simulink model "sampleModel1602"  (R2023a)
settings: Solver=VariableStepAuto  StartTime=0.0  StopTime=10.0  RelTol=1e-3
libraries: hdlsllib x5, simulink x1
settings Model: Creator=user1  LastModifiedBy=user1

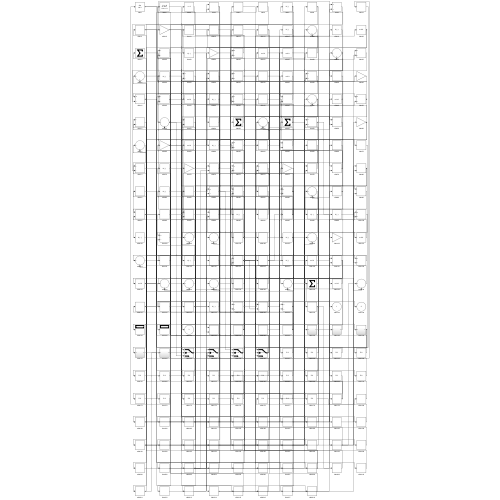
[thumbnail: Simulink's stored preview of the top-level diagram]
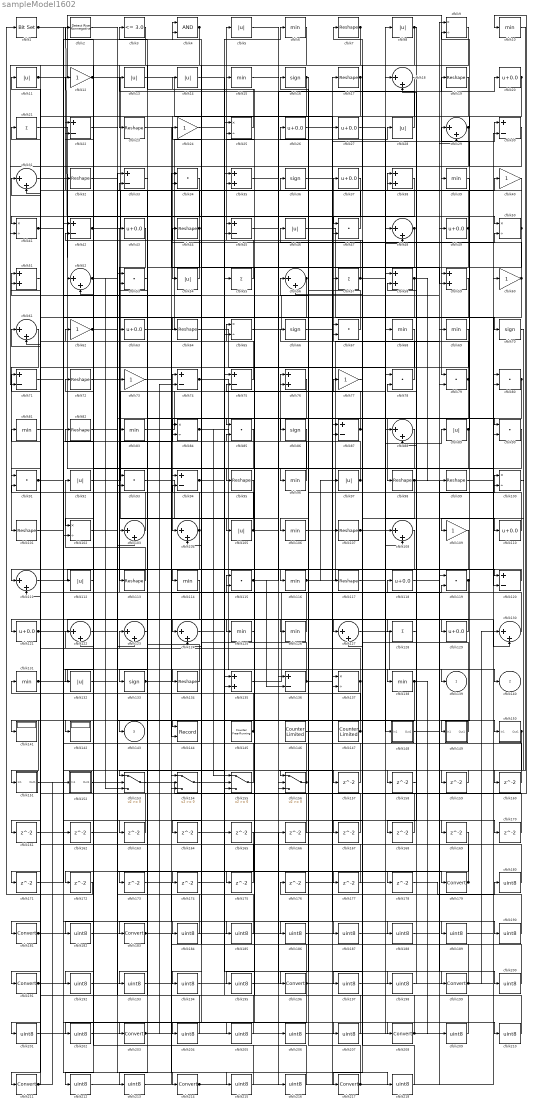
== system sampleModel1602 ==
  cfblk1 : simulink/Logic and Bit Operations/Bit Set  iBit=0
      settings: LibrarySourceBlock=|
      | hdlsllib/Logic and Bit
      | Operations/Bit Set
  cfblk{6,10,15,39,68..69,81,83,96,106,114,116,125..126,131,138} (16 alike) : MinMax
  cfblk{9,25,41,50,65,84,100,102,137} (9 alike) : Product  Inputs=*/  RndMeth=Zero  SaturateOnIntegerOverflow=on
  cfblk{7,17,19,23,32,44,64,72,82,95,98..99,101,107,113,117,134} (17 alike) : Reshape
  cfblk{18,29,31,48,52,56,61,88,103..104,108,111,122..124,127,130} (17 alike) : Sum  Inputs=|++
  cfblk{5,8,11,13..14,28,46,54,89,92,97,105,112,132} (14 alike) : Abs  SaturateOnIntegerOverflow=off
  cfblk{12,24,40,60,62,73,77,109} (8 alike) : Gain
  cfblk{20,26..27,37,43,49,63,110,118,121,129} (11 alike) : Bias  Bias=0.0  SaturateOnIntegerOverflow=off
  cfblk{34,47,53,67,78..80,85,90..91,93,115,119} (13 alike) : DotProduct  OutDataTypeStr=Inherit: Inherit via internal rule
  cfblk{22,30,33,42,45,71,74..75,87,94,120,136} (12 alike) : Sum  Inputs=+-
  cfblk{21,55,57,128} (4 alike) : Sum  Inputs=+
  cfblk{16,36,66,70,86,133} (6 alike) : Signum
  cfblk{35,38,51,58..59,76,135} (7 alike) : Sum
  cfblk141 : Display
  cfblk142 : Display
  cfblk144 : Record  FileSettingsInternal="{\"entries\":[{\"content\":{\"excelSettings\":{\"content\":{},\"type\":\"Streamout.ExcelSettings\"}},\"type\":\"Streamout.FileSettingStorage\",\"uuid\":\"\"}],\"packageUris\":[\"http:\\/\\/schema.mathworks.com\\/mf0\\/streamout_blocks\\/R2020a\"],\"version\":\"1.0\"}"  Layout=[1 1]  SignalsInternal="{\"entries\":[{\"content\":{\"signals\":[{\"content\":{\"blockPath\":[],\"dimensions\":[1],\"domain\":\"\",\"lineColor\":\"#a2142f\",\"plots\":[1],\"port\":1,\"signalID\":2228,\"signalName\":\"XY Graph:1\"},\"type\":\"RecordBlkView.Signal\",\"uuid\":\"\"},{\"content\":{\"blockPath\":[],\"dimensions\":[1],\"domain\":\"\",\"lineColor\":\"#139fff\",\"plots\":[1],\"port\":2,\"signalID\":2231,\"signalName\":\"XY Graph:2\"},\"type\":\"RecordBlkView.Signal\",\"uuid\":\"\"}]},\"type\":\"RecordBlkView.InputSignals\",\"uuid\":\"\"}],\"packageUris\":[\"http:\\/\\/schema.mathworks.com\\/mf0\\/streamout_blocks\\/R2020a\"],\"version\":\"1.0\"}"  VisualizationBindings="{\"xyplotplugin\":{\"info\":[{\"series\":[{\"bindingParametersList\":[{\"parameter\":\"X-Axis\",\"signalID\":2228,\"signalName\":\"XY Graph:1\"},{\"parameter\":\"Y-Axis\",\"signalID\":2231,\"signalName\":\"XY Graph:2\"}],\"seriesID\":22557}],\"subplotID\":1}]}}"  CompatibilityTag=XY  st=-1
  cfblk145 : hdlsllib/Sources/Counter Free-Running  NumBits=16  tsamp=-1
  cfblk146 : hdlsllib/Sources/Counter Limited  uplimit=7  tsamp=-1
  cfblk147 : hdlsllib/Sources/Counter Limited  uplimit=7  tsamp=-1
  cfblk148 : Subsystem
      settings: LibrarySourceBlock=|
      | hdlsllib/Ports &
      | Subsystems/Subsystem
  cfblk149 : Subsystem
      settings: LibrarySourceBlock=|
      | hdlsllib/Ports &
      | Subsystems/Subsystem
  cfblk150 : Subsystem
      settings: LibrarySourceBlock=|
      | hdlsllib/Ports &
      | Subsystems/Subsystem
  cfblk151 : Subsystem
      settings: LibrarySourceBlock=|
      | hdlsllib/Ports &
      | Subsystems/Subsystem
  cfblk152 : Subsystem
      settings: LibrarySourceBlock=|
      | hdlsllib/Ports &
      | Subsystems/Subsystem
  cfblk{153..156} (4 alike) : Switch  SaturateOnIntegerOverflow=off  InputSameDT=off
  cfblk{157..178} (22 alike) : Delay  SampleTime=1
  cfblk{179,181,183,191,196,199,203,208,211,214,217} (11 alike) : DataTypeConversion  SaturateOnIntegerOverflow=off  RndMeth=Floor
  cfblk{180,182,184..190,192..195,197..198,200..202,204..207,209..210,212..213,215..216,218} (29 alike) : DataTypeConversion  OutDataTypeStr=uint8  SaturateOnIntegerOverflow=off  RndMeth=Floor
  cfblk2 : hdlsllib/Logic and Bit Operations/Detect Rise Nonnegative  vinit=0  OutDataTypeStr=boolean
  cfblk3 : hdlsllib/Logic and Bit Operations/Compare To Constant  relop=<=  const=3.0  OutDataTypeStr=boolean
  cfblk4 : Logic  AllPortsSameDT=off  OutDataTypeStr=boolean
  cfblk139 : Outport  VectorParamsAs1DForOutWhenUnconnected=off
  cfblk140 : Outport  Port=2  VectorParamsAs1DForOutWhenUnconnected=off
  cfblk143 : Outport  Port=3  VectorParamsAs1DForOutWhenUnconnected=off
  wires:
  cfblk33/1 -> cfblk203/1
  cfblk127/1 -> cfblk139/1
  cfblk8/1 -> cfblk167/1, cfblk168/1
  cfblk135/1 -> cfblk118/1
  cfblk84/1 -> cfblk120/1, cfblk155/1
  cfblk119/1 -> cfblk131/1, cfblk174/1, cfblk201/1
  cfblk117/1 -> cfblk89/1
  cfblk57/1 -> cfblk5/1, cfblk110/1
  cfblk74/1 -> cfblk140/1, cfblk4/1
  cfblk12/1 -> cfblk105/1, cfblk100/2
  cfblk42/1 -> cfblk38/1, cfblk102/1
  cfblk53/1 -> cfblk183/1
  cfblk52/1 -> cfblk123/2, cfblk153/3
  cfblk63/1 -> cfblk28/1
  cfblk21/1 -> cfblk96/1
  cfblk126/1 -> cfblk43/1
  cfblk11/1 -> cfblk79/1, cfblk155/3
  cfblk43/1 -> cfblk113/1
  cfblk64/1 -> cfblk148/1(In1)
  cfblk19/1 -> cfblk54/1
  cfblk38/1 -> cfblk126/1
  cfblk61/1 -> cfblk101/1
  cfblk20/1 -> cfblk41/1, cfblk39/1
  cfblk70/1 -> cfblk109/1
  cfblk97/1 -> cfblk74/1, cfblk83/1
  cfblk78/1 -> cfblk37/1
  cfblk125/1 -> cfblk45/1
  cfblk24/1 -> cfblk55/1
  cfblk96/1 -> cfblk76/1
  cfblk154/1 -> cfblk199/1
  cfblk89/1 -> cfblk29/1, cfblk94/1
  cfblk7/1 -> cfblk114/1, cfblk173/1
  cfblk69/1 -> cfblk181/1
  cfblk128/1 -> cfblk58/2
  cfblk39/1 -> cfblk149/1(In1)
  cfblk1/1 -> cfblk52/1, cfblk65/2
  cfblk79/1 -> cfblk98/1, cfblk26/1, cfblk66/1
  cfblk129/1 -> cfblk125/1
  cfblk9/1 -> cfblk23/1
  cfblk76/1 -> cfblk104/1
  cfblk48/1 -> cfblk95/1, cfblk204/1
  cfblk35/1 -> cfblk208/1
  cfblk121/1 -> cfblk124/1, cfblk84/2, cfblk4/2
  cfblk146/1 -> cfblk27/1
  cfblk95/1 -> cfblk103/1
  cfblk40/1 -> cfblk38/2
  cfblk67/1 -> cfblk16/1
  cfblk14/1 -> cfblk179/1
  cfblk31/1 -> cfblk47/1
  cfblk80/1 -> cfblk153/1, cfblk158/1
  cfblk150/1(Out1) -> cfblk195/1, cfblk213/1
  cfblk108/1 -> cfblk191/1
  cfblk2/1 -> cfblk103/2
  cfblk4/1 -> cfblk141/1, cfblk192/1
  cfblk138/1 -> cfblk155/2, cfblk209/1
  cfblk111/1 -> cfblk116/1
  cfblk107/1 -> cfblk129/1, cfblk197/1
  cfblk149/1(Out1) -> cfblk56/2
  cfblk94/1 -> cfblk24/1, cfblk6/1
  cfblk60/1 -> cfblk46/1, cfblk87/2, cfblk171/1
  cfblk37/1 -> cfblk91/1
  cfblk47/1 -> cfblk12/1
  cfblk72/1 -> cfblk90/1
  cfblk105/1 -> cfblk136/1, cfblk72/1
  cfblk102/1 -> cfblk128/1
  cfblk147/1 -> cfblk44/1, cfblk84/1
  cfblk17/1 -> cfblk45/2, cfblk143/1
  cfblk93/1 -> cfblk156/2
  cfblk115/1 -> cfblk20/1, cfblk136/2, cfblk130/2, cfblk178/1, cfblk198/1
  cfblk75/1 -> cfblk31/2
  cfblk28/1 -> cfblk13/1
  cfblk136/1 -> cfblk19/1, cfblk51/2
  cfblk22/1 -> cfblk67/2
  cfblk30/1 -> cfblk59/1
  cfblk27/1 -> cfblk70/1
  cfblk50/1 -> cfblk7/1, cfblk135/2
  cfblk153/1 -> cfblk10/1
  cfblk131/1 -> cfblk134/1, cfblk57/1
  cfblk92/1 -> cfblk17/1
  cfblk123/1 -> cfblk93/1
  cfblk56/1 -> cfblk104/2, cfblk64/1, cfblk144/2
  cfblk26/1 -> cfblk50/1
  cfblk44/1 -> cfblk21/1, cfblk193/1
  cfblk25/1 -> cfblk3/1
  cfblk66/1 -> cfblk30/1
  cfblk113/1 -> cfblk92/1
  cfblk116/1 -> cfblk9/1, cfblk97/1
  cfblk77/1 -> cfblk217/1
  cfblk134/1 -> cfblk63/1
  cfblk88/1 -> cfblk196/1
  cfblk86/1 -> cfblk133/1
  cfblk118/1 -> cfblk100/1
  cfblk73/1 -> cfblk50/2
  cfblk54/1 -> cfblk42/2
  cfblk106/1 -> cfblk48/1
  cfblk130/1 -> cfblk71/1
  cfblk46/1 -> cfblk120/2
  cfblk109/1 -> cfblk156/3
  cfblk91/1 -> cfblk138/1, cfblk153/2
  cfblk99/1 -> cfblk90/2
  cfblk13/1 -> cfblk107/1
  cfblk3/1 -> cfblk41/2
  cfblk58/1 -> cfblk86/1, cfblk99/1
  cfblk29/1 -> cfblk71/2, cfblk9/2, cfblk142/1
  cfblk103/1 -> cfblk81/1
  cfblk155/1 -> cfblk82/1
  cfblk65/1 -> cfblk29/2
  cfblk34/1 -> cfblk211/1
  cfblk145/1 -> cfblk62/1, cfblk115/1
  cfblk87/1 -> cfblk65/1, cfblk127/1
  cfblk112/1 -> cfblk22/1
  cfblk55/1 -> cfblk2/1
  cfblk156/1 -> cfblk32/1, cfblk22/2
  cfblk62/1 -> cfblk144/1, cfblk40/1
  cfblk49/1 -> cfblk25/2, cfblk85/1
  cfblk120/1 -> cfblk111/1
  cfblk16/1 -> cfblk106/1, cfblk132/1
  cfblk122/1 -> cfblk214/1
  cfblk83/1 -> cfblk8/1
  cfblk110/1 -> cfblk76/2
  cfblk137/1 -> cfblk151/1(In1), cfblk51/1
  cfblk51/1 -> cfblk111/2
  cfblk104/1 -> cfblk121/1, cfblk94/2
  cfblk41/1 -> cfblk112/1, cfblk61/2
  cfblk124/1 -> cfblk135/1
  cfblk98/1 -> cfblk127/2, cfblk200/1
  cfblk133/1 -> cfblk150/1(In1), cfblk119/2
  cfblk23/1 -> cfblk59/2
  cfblk45/1 -> cfblk157/1
  cfblk157/1 -> cfblk42/1
  cfblk158/1 -> cfblk78/2
  cfblk10/1 -> cfblk159/1
  cfblk159/1 -> cfblk156/1
  cfblk100/1 -> cfblk160/1
  cfblk160/1 -> cfblk75/2
  cfblk59/1 -> cfblk161/1
  cfblk71/1 -> cfblk162/1
  cfblk162/1 -> cfblk93/2
  cfblk81/1 -> cfblk163/1
  cfblk163/1 -> cfblk52/2
  cfblk6/1 -> cfblk164/1
  cfblk164/1 -> cfblk67/1
  cfblk166/1 -> cfblk91/2
  cfblk167/1 -> cfblk123/1
  cfblk168/1 -> cfblk47/2
  cfblk82/1 -> cfblk169/1
  cfblk148/1(Out1) -> cfblk170/1
  cfblk170/1 -> cfblk58/1
  cfblk171/1 -> cfblk102/2
  cfblk114/1 -> cfblk172/1
  cfblk172/1 -> cfblk1/1
  cfblk90/1 -> cfblk175/1
  cfblk175/1 -> cfblk31/1
  cfblk176/1 -> cfblk48/2
  cfblk132/1 -> cfblk177/1
  cfblk177/1 -> cfblk25/1
  cfblk179/1 -> cfblk115/2, cfblk137/1
  cfblk178/1 -> cfblk180/1
  cfblk180/1 -> cfblk14/1
  cfblk181/1 -> cfblk137/2, cfblk73/1
  cfblk85/1 -> cfblk182/1
  cfblk182/1 -> cfblk69/1
  cfblk183/1 -> cfblk75/1, cfblk218/1
  cfblk101/1 -> cfblk184/1
  cfblk184/1 -> cfblk53/1
  cfblk173/1 -> cfblk185/1
  cfblk185/1 -> cfblk53/2
  cfblk18/1 -> cfblk186/1
  cfblk186/1 -> cfblk49/1
  cfblk32/1 -> cfblk187/1
  cfblk187/1 -> cfblk18/1
  cfblk174/1 -> cfblk188/1
  cfblk188/1 -> cfblk18/2
  cfblk36/1 -> cfblk189/1
  cfblk189/1 -> cfblk80/1
  cfblk152/1(Out1) -> cfblk190/1
  cfblk190/1 -> cfblk36/1
  cfblk191/1 -> cfblk166/1, cfblk165/1, cfblk215/1
  cfblk192/1 -> cfblk108/1
  cfblk193/1 -> cfblk108/2
  cfblk68/1 -> cfblk194/1
  cfblk194/1 -> cfblk80/2
  cfblk195/1 -> cfblk68/1
  cfblk196/1 -> cfblk124/2, cfblk212/1
  cfblk197/1 -> cfblk88/1
  cfblk198/1 -> cfblk88/2
  cfblk199/1 -> cfblk60/1, cfblk130/1, cfblk56/1
  cfblk200/1 -> cfblk154/1
  cfblk201/1 -> cfblk154/2
  cfblk165/1 -> cfblk202/1
  cfblk202/1 -> cfblk154/3
  cfblk203/1 -> cfblk87/1, cfblk74/2, cfblk78/1
  cfblk204/1 -> cfblk33/1
  cfblk169/1 -> cfblk205/1
  cfblk205/1 -> cfblk33/2
  cfblk15/1 -> cfblk206/1
  cfblk206/1 -> cfblk79/2
  cfblk151/1(Out1) -> cfblk207/1
  cfblk207/1 -> cfblk15/1
  cfblk208/1 -> cfblk85/2, cfblk61/1
  cfblk209/1 -> cfblk35/1
  cfblk161/1 -> cfblk210/1
  cfblk210/1 -> cfblk35/2
  cfblk211/1 -> cfblk11/1, cfblk152/1(In1)
  cfblk212/1 -> cfblk34/1
  cfblk213/1 -> cfblk34/2
  cfblk214/1 -> cfblk30/2, cfblk117/1
  cfblk215/1 -> cfblk122/1
  cfblk5/1 -> cfblk216/1
  cfblk216/1 -> cfblk122/2
  cfblk217/1 -> cfblk176/1, cfblk119/1
  cfblk218/1 -> cfblk77/1

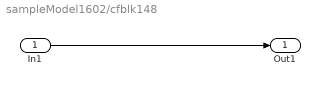
== system sampleModel1602/cfblk148 ==
  In1 : Inport
  Out1 : Outport
  wires:
  In1/1 -> Out1/1

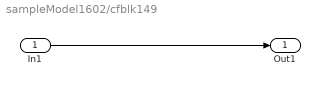
== system sampleModel1602/cfblk149 ==
  In1 : Inport
  Out1 : Outport
  wires:
  In1/1 -> Out1/1

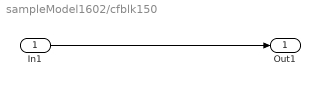
== system sampleModel1602/cfblk150 ==
  In1 : Inport
  Out1 : Outport
  wires:
  In1/1 -> Out1/1

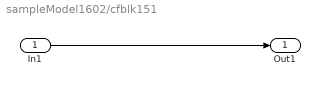
== system sampleModel1602/cfblk151 ==
  In1 : Inport
  Out1 : Outport
  wires:
  In1/1 -> Out1/1

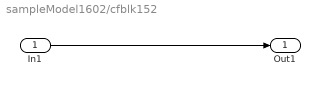
== system sampleModel1602/cfblk152 ==
  In1 : Inport
  Out1 : Outport
  wires:
  In1/1 -> Out1/1
